simulink model "sedemo_ethernet"  (Simulink 7.5)
settings: Solver=VariableStepDiscrete  StartTime=0.0  StopTime=10.0  MaxStep=inf  RelTol=1e-3
PreLoadFcn:
  | MACInputSize = 25;
  | warning('off','MATLAB:divideByZero');
undefined symbols (not defined in the file or in its folder): des_subsystemblock, des_subsysteminport, des_subsystemoutport, des_subsystemsupportblock
libraries: simeventsrouting1 x30, simeventstranslate1 x26, simeventsattributes2 x16, simeventssink1 x13, simeventsserver1 x13, simeventsgenerators1 x11, simeventssignalmanage1 x9, simeventsgates1 x6, simeventsqueue1 x3, simeventsinfo x1
(part 1 of 5)
CloseFcn:
  | clear MACInputSize;
  | clear tout;
settings Model: Creator=The MathWorks Inc.
settings DataIOCC: SaveOutput=off  SaveTime=off
settings DebuggingCC: AlgebraicLoopMsg=error  SolverPrmCheckMsg=none  StrictBusMsg=Warning
settings SimEventsCC: propDiagAttribOutput=1  propDiagFcnCallOutput=1  propDiagStatOutput=0

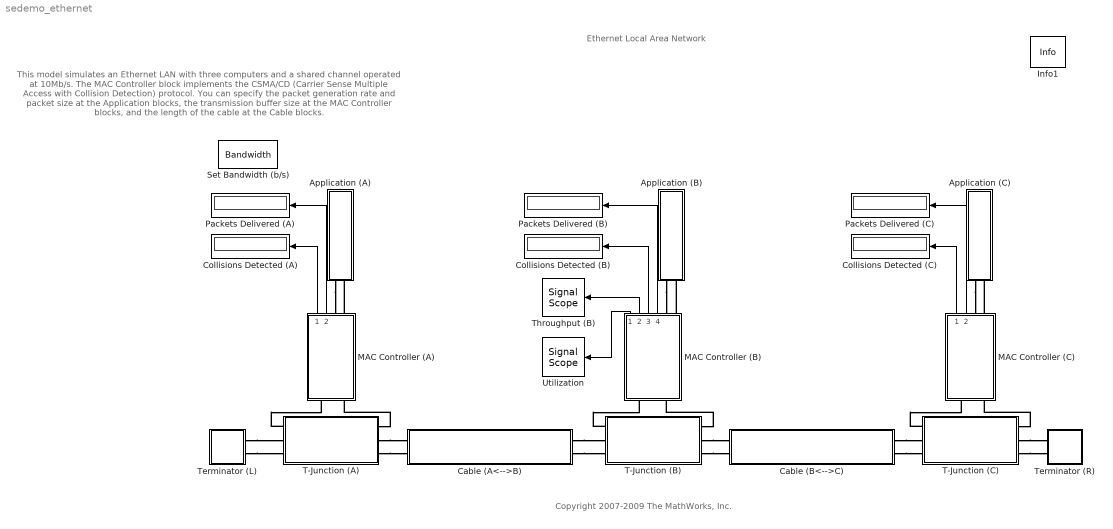
== system sedemo_ethernet ==
  note: Ethernet Local Area Network
  note: This model simulates an Ethernet LAN with three computers and a shared channel operated at 10Mb/s. The MAC Controller block implements the CSMA/CD
      | (Carrier Sense Multiple Access with Collision Detection) protocol. You can specify the packet generation rate and packet size at the Application blocks, the
      | transmission buffer size at the MAC Controller blocks, and the length of the cable at the Cable blocks.
  note: Copyright 2007-2009 The MathWorks, Inc.
  Application (A) : Subsystem  mask(Application){PacketRate=100, MinPacketSize=64, MaxPacketSize=1500, RandomSeed=678}
      mask prompts: PacketRate "Rate of packet generation (packets/s):"; MinPacketSize "Minimum packet size (bytes):"; MaxPacketSize "Maximum packet size (bytes):"; RandomSeed "Initial seed:"
      mask help: Model the generation and consumption of Ethernet data packets. Packet generation is modeled as a Poisson process. Packet size is uniformly distributed. You can specify the packet generation rate, minimum packet size and maximum packet size.
  Application (B) : Subsystem  mask(Application){PacketRate=100, MinPacketSize=64, MaxPacketSize=1500, RandomSeed=47984}
      mask prompts: PacketRate "Rate of packet generation (packets/s):"; MinPacketSize "Minimum packet size (bytes):"; MaxPacketSize "Maximum packet size (bytes):"; RandomSeed "Initial seed:"
      mask help: Model the generation and consumption of Ethernet data packets. Packet generation is modeled as a Poisson process. Packet size is uniformly distributed. You can specify the packet generation rate, minimum packet size and maximum packet size.
  Application (C) : Subsystem  mask(Application){PacketRate=100, MinPacketSize=64, MaxPacketSize=1500, RandomSeed=327278}
      mask prompts: PacketRate "Rate of packet generation (packets/s):"; MinPacketSize "Minimum packet size (bytes):"; MaxPacketSize "Maximum packet size (bytes):"; RandomSeed "Initial seed:"
      mask help: Model the generation and consumption of Ethernet data packets. Packet generation is modeled as a Poisson process. Packet size is uniformly distributed. You can specify the packet generation rate, minimum packet size and maximum packet size.
  Cable (A<-->B) : Subsystem  mask(Cable){CableLength=100}
      mask prompts: CableLength "Length (m):"
      mask help: Model the physical connection between two network terminals and the corresponding propagation delay during data transmission. You can specify the length of the cable.
  Cable (B<-->C) : Subsystem  mask(Cable){CableLength=200}
      mask prompts: CableLength "Length (m):"
      mask help: Model the physical connection between two network terminals and the corresponding propagation delay during data transmission. You can specify the length of the cable.
  "Collisions Detected (A) " : Display
  Collisions Detected (B) : Display
  Collisions Detected (C) : Display
  Info1 : simeventsinfo/Info  SystemSampleTime=-1
  MAC Controller (A) : Subsystem  mask(MAC Controller){SrcAddress=1, MACInputSize=25}
      mask prompts: SrcAddress "Source address:"; MACInputSize "Size of transmission buffer (packets):"
      mask help: Model an Ethernet controller that implements the CSMA/CD (Carrier Sense Multiple Access with Collision Detection) protocol and the binary exponential backoff algorithm. You can specify the source address of the packet and the size of the transmission buffer.
  MAC Controller (B) : Subsystem  mask(MAC Controller){SrcAddress=2, MACInputSize=25}
      mask prompts: SrcAddress "Source address:"; MACInputSize "Size of transmission buffer (packets):"
      mask help: Model an Ethernet controller that implements the CSMA/CD (Carrier Sense Multiple Access with Collision Detection) protocol and the binary exponential backoff algorithm. You can specify the source address of the packet and the size of the transmission buffer.
  MAC Controller (C) : Subsystem  mask(MAC Controller){SrcAddress=3, MACInputSize=25}
      mask prompts: SrcAddress "Source address:"; MACInputSize "Size of transmission buffer (packets):"
      mask help: Model an Ethernet controller that implements the CSMA/CD (Carrier Sense Multiple Access with Collision Detection) protocol and the binary exponential backoff algorithm. You can specify the source address of the packet and the size of the transmission buffer.
  Packets Delivered (A) : Display
  Packets Delivered (B) : Display
  Packets Delivered (C) : Display
  Set Bandwidth (b/s) : DataStoreMemory  DataStoreName=Bandwidth  InitialValue=1e7  OutDataType=sfix(16)  OutScaling=2^0
  T-Junction (A) : Subsystem
      mask Type: T-Junction
      mask Description: Connect cables from adjacent remote terminals to the local Ethernet adapter.
  T-Junction (B) : Subsystem
      mask Type: T-Junction
      mask Description: Connect cables from adjacent remote terminals to the local Ethernet adapter.
  T-Junction (C) : Subsystem
      mask Type: T-Junction
      mask Description: Connect cables from adjacent remote terminals to the local Ethernet adapter.
  Terminator (L) : Subsystem
      mask Type: Terminator
      mask Description: End an Ethernet connection.
  Terminator (R) : Subsystem
      mask Type: Terminator
      mask Description: End an Ethernet connection.
  Throughput (B) : simeventssink1/Signal Scope  Priority=1  SystemSampleTime=-1  PlotType=Stair  InputType=Signal  NumInputs=1  AttributeNameY=Count  XInputOptionSignal=Event time  XInputOptionEntity=Event time  AttributeNameX=Count  EnableEntityOutport=on  XMin=0  XMax=20  XLimitExceededOption=Stretch axis limits  YLimitExceededOption=Stretch axis limits  AxisGrid=on  AxisLegend=off  LineDisables=""  LineColors=b  LineStyles=-  LineMarkers=None  OpenScopeAtSimStart=on  Title=Throughput (kbps)  YLabel=""  XLabel=Time  FigurePosition=[635 446 386 253]  AxisZoom=off  DataStoreOption=Unlimited  DataPointsLimit=10000  StatNumberArrived=Off  ShowCountPlotted=off  ShowToolbar=on
      settings: YMin=0  YMax=1000
  Utilization : simeventssink1/Signal Scope  Priority=1  SystemSampleTime=-1  PlotType=Stair  InputType=Signal  NumInputs=1  AttributeNameY=Count  XInputOptionSignal=Event time  XInputOptionEntity=Event time  AttributeNameX=Count  EnableEntityOutport=on  XMin=0  XMax=20  XLimitExceededOption=Stretch axis limits  YLimitExceededOption=Stretch axis limits  AxisGrid=on  AxisLegend=off  LineDisables=""  LineColors=[1 0 0]  LineStyles=-  LineMarkers=None  OpenScopeAtSimStart=on  Title=Channel Utilization  YLabel=""  XLabel=Time  FigurePosition=[635 120 387 253]  AxisZoom=off  DataStoreOption=Unlimited  DataPointsLimit=10000  StatNumberArrived=Off  ShowCountPlotted=off  ShowToolbar=on
      settings: YMin=0  YMax=0.5
  wires:
  MAC Controller (A)/1(#collision) -> "Collisions Detected (A) "/1
  MAC Controller (A)/2(#success) -> Packets Delivered (A)/1
  MAC Controller (B)/3(#collision) -> Collisions Detected (B)/1
  MAC Controller (B)/4(#success) -> Packets Delivered (B)/1
  MAC Controller (B)/1(utilization) -> Utilization/1
  MAC Controller (C)/1(#collision) -> Collisions Detected (C)/1
  MAC Controller (C)/2(#success) -> Packets Delivered (C)/1
  MAC Controller (B)/2(throughput) -> Throughput (B)/1
  connections:
  Cable (B<-->C)/RConn2 -- T-Junction (C)/LConn3
  Cable (B<-->C)/RConn1 -- T-Junction (C)/LConn2
  T-Junction (B)/RConn3 -- Cable (B<-->C)/LConn2
  T-Junction (B)/RConn2 -- Cable (B<-->C)/LConn1
  T-Junction (C)/LConn1 -- MAC Controller (C)/LConn1
  T-Junction (C)/RConn1 -- MAC Controller (C)/LConn2
  T-Junction (C)/RConn2 -- Terminator (R)/LConn1
  T-Junction (C)/RConn3 -- Terminator (R)/LConn2
  MAC Controller (C)/RConn2 -- Application (C)/RConn2
  Application (C)/RConn1 -- MAC Controller (C)/RConn1
  Application (A)/RConn1 -- MAC Controller (A)/RConn1
  Cable (A<-->B)/RConn2 -- T-Junction (B)/LConn3
  Cable (A<-->B)/RConn1 -- T-Junction (B)/LConn2
  T-Junction (B)/LConn1 -- MAC Controller (B)/LConn1
  Application (B)/RConn1 -- MAC Controller (B)/RConn1
  MAC Controller (B)/RConn2 -- Application (B)/RConn2
  T-Junction (B)/RConn1 -- MAC Controller (B)/LConn2
  MAC Controller (A)/RConn2 -- Application (A)/RConn2
  Terminator (L)/LConn2 -- T-Junction (A)/LConn3
  Terminator (L)/LConn1 -- T-Junction (A)/LConn2
  T-Junction (A)/RConn3 -- Cable (A<-->B)/LConn2
  T-Junction (A)/RConn2 -- Cable (A<-->B)/LConn1
  T-Junction (A)/RConn1 -- MAC Controller (A)/LConn2
  T-Junction (A)/LConn1 -- MAC Controller (A)/LConn1

== system sedemo_ethernet/Application (A) ==
  note: Network Application
  Compute comm delay : Subsystem  LoadFcn=des_subsystemblock(gcb, 'load');  InitFcn=des_subsystemblock(gcb, 'init');  StartFcn=des_subsystemblock(gcb, 'start');  StopFcn=des_subsystemblock(gcb, 'stop');
      settings: CopyFcn=des_subsystemblock(gcb, 'copy');  DeleteFcn=des_subsystemblock(gcb, 'delete');  UndoDeleteFcn=des_subsystemblock(gcb, 'undodelete');  ModelCloseFcn=des_subsystemblock(gcb, 'modelclose');  PreSaveFcn=des_subsystemblock(gcb, 'presave');  NameChangeFcn=des_subsystemblock(gcb, 'namechange');  ParentCloseFcn=des_subsystemblock(gcb, 'parentclose');  ErrorFcn=des_error_redirect
  Data User : simeventssink1/Entity Sink  Priority=1  SystemSampleTime=-1  AvailableForArrivals=on  StatNumberArrived=Off
  Event-Based Random Number1 : simeventsgenerators1/Signal Generators/Event-Based Random Number  SystemSampleTime=-1  distribution=Uniform  meanExp=1/PacketRate  minUnif=MinPacketSize*8  maxUnif=MaxPacketSize*8  pOneBern=0.25  pSuccessBino=0.5  numTrialBino=1  meanNorm=0  stdNorm=1  minTri=1  maxTri=3  modeTri=2  thresholdLogn=0  scaleLogn=1  shapeLogn=1  pSuccessGeo=0.5  meanPoiss=1  thresholdLogl=0  scaleLogl=1  thresholdGam=0  scaleGam=1  shapeGam=1  minBeta=0  maxBeta=1  shape1Beta=1  shape2Beta=1  minUnid=0  maxUnid=1  numValueUnid=2  thresholdWbl=0  scaleWbl=1  shapeWbl=1  valueVecCont=[0 1]  cdfVecCont=[0 1]  valueVecDisc=[0 1]  probVecDisc=[0.5 0.5]  seed=RandomSeed+12345  IsProcessed=on  isConnected=1
  Event-Based Random Number2 : simeventsgenerators1/Signal Generators/Event-Based Random Number  SystemSampleTime=-1  distribution=Exponential  meanExp=1/PacketRate  minUnif=MinPacketSize  maxUnif=MaxPacketSize  pOneBern=0.25  pSuccessBino=0.5  numTrialBino=1  meanNorm=0  stdNorm=1  minTri=1  maxTri=3  modeTri=2  thresholdLogn=0  scaleLogn=1  shapeLogn=1  pSuccessGeo=0.5  meanPoiss=1  thresholdLogl=0  scaleLogl=1  thresholdGam=0  scaleGam=1  shapeGam=1  minBeta=0  maxBeta=1  shape1Beta=1  shape2Beta=1  minUnid=0  maxUnid=1  numValueUnid=2  thresholdWbl=0  scaleWbl=1  shapeWbl=1  valueVecCont=[0 1]  cdfVecCont=[0 1]  valueVecDisc=[0 1]  probVecDisc=[0.5 0.5]  seed=RandomSeed  IsProcessed=on  isConnected=1
  Set Attribute (Set packet size and comm delay) : simeventsattributes2/Set Attribute  Priority=1  DialogController=des_ddg_create  DialogControllerArgs=DataTag9  SystemSampleTime=-1  AttributeFrom=Signal port|Signal port  AttributeName=PacketSize|ServiceTime  AttributeTreatAsVector=1|1  AttributeValue=0.1|0  AttributeCreate=on  StatNumberDeparted=On  EvaluatedAttributeValue={[];[]}
  Signal Latch : simeventssignalmanage1/Signal Latch  Priority=1  SystemSampleTime=-1  InitialMemoryValue=512  WriteMemoryUpon=Change in signal from port wvc  MemoryWriteEdgeOption=Rising  SpecifyWriteEventPriority=off  PriorityMemoryWrite=7100  ReadMemoryUpon=Write to memory event  MemoryReadEdgeOption=Falling  SpecifyReadEventPriority=on  PriorityMemoryRead=7000  ReportMemoryState=off  ReportMemoryUponWrite=off  ReportMemoryUponRead=on
  Time-Based Entity Generator : simeventsgenerators1/Entity Generators/Time-Based Entity Generator  Priority=1  DialogController=des_ddg_create  DialogControllerArgs=DataTag12  SystemSampleTime=-1  GenerateEntitiesUpon=Intergeneration time from port t  Distribution=Constant  Minimum=0  Maximum=1  Mean=1/PacketRate  InitialSeed=2  Period=0.01  PriorityEntityGeneration=300  GenerateEntityAtSimulationStart=off  ResponseWhenBlocked=Pause generation  ResponseWhenUnblocked=Immediate restart  EntityType=Standard  StatNumberDeparted=Off  StatPendingEntity=Off  StatAverageIntergenerationTime=Off
  OUT : PMIOPort  Port=1  Side=Right
  IN : PMIOPort  Port=2  Side=Right
  wires:
  Compute comm delay/1(delay) -> Set Attribute (Set packet size and comm delay)/2
  Signal Latch/1 -> Compute comm delay/1(size), Set Attribute (Set packet size and comm delay)/1
  Event-Based Random Number1/1 -> Signal Latch/2
  Set Attribute (Set packet size and comm delay)/1 -> Signal Latch/1
  Event-Based Random Number2/1 -> Time-Based Entity Generator/1
  connections:
  IN/RConn1 -- Data User/LConn1
  OUT/RConn1 -- Set Attribute (Set packet size and comm delay)/RConn1
  Time-Based Entity Generator/RConn1 -- Set Attribute (Set packet size and comm delay)/LConn1

== system sedemo_ethernet/Application (B) ==
  note: Network Application
  Compute comm delay : Subsystem  LoadFcn=des_subsystemblock(gcb, 'load');  InitFcn=des_subsystemblock(gcb, 'init');  StartFcn=des_subsystemblock(gcb, 'start');  StopFcn=des_subsystemblock(gcb, 'stop');
      settings: CopyFcn=des_subsystemblock(gcb, 'copy');  DeleteFcn=des_subsystemblock(gcb, 'delete');  UndoDeleteFcn=des_subsystemblock(gcb, 'undodelete');  ModelCloseFcn=des_subsystemblock(gcb, 'modelclose');  PreSaveFcn=des_subsystemblock(gcb, 'presave');  NameChangeFcn=des_subsystemblock(gcb, 'namechange');  ParentCloseFcn=des_subsystemblock(gcb, 'parentclose');  ErrorFcn=des_error_redirect
  Data User : simeventssink1/Entity Sink  Priority=1  SystemSampleTime=-1  AvailableForArrivals=on  StatNumberArrived=Off
  Event-Based Random Number1 : simeventsgenerators1/Signal Generators/Event-Based Random Number  SystemSampleTime=-1  distribution=Uniform  meanExp=1/PacketRate  minUnif=MinPacketSize*8  maxUnif=MaxPacketSize*8  pOneBern=0.25  pSuccessBino=0.5  numTrialBino=1  meanNorm=0  stdNorm=1  minTri=1  maxTri=3  modeTri=2  thresholdLogn=0  scaleLogn=1  shapeLogn=1  pSuccessGeo=0.5  meanPoiss=1  thresholdLogl=0  scaleLogl=1  thresholdGam=0  scaleGam=1  shapeGam=1  minBeta=0  maxBeta=1  shape1Beta=1  shape2Beta=1  minUnid=0  maxUnid=1  numValueUnid=2  thresholdWbl=0  scaleWbl=1  shapeWbl=1  valueVecCont=[0 1]  cdfVecCont=[0 1]  valueVecDisc=[0 1]  probVecDisc=[0.5 0.5]  seed=RandomSeed+12345  IsProcessed=on  isConnected=1
  Event-Based Random Number2 : simeventsgenerators1/Signal Generators/Event-Based Random Number  SystemSampleTime=-1  distribution=Exponential  meanExp=1/PacketRate  minUnif=MinPacketSize  maxUnif=MaxPacketSize  pOneBern=0.25  pSuccessBino=0.5  numTrialBino=1  meanNorm=0  stdNorm=1  minTri=1  maxTri=3  modeTri=2  thresholdLogn=0  scaleLogn=1  shapeLogn=1  pSuccessGeo=0.5  meanPoiss=1  thresholdLogl=0  scaleLogl=1  thresholdGam=0  scaleGam=1  shapeGam=1  minBeta=0  maxBeta=1  shape1Beta=1  shape2Beta=1  minUnid=0  maxUnid=1  numValueUnid=2  thresholdWbl=0  scaleWbl=1  shapeWbl=1  valueVecCont=[0 1]  cdfVecCont=[0 1]  valueVecDisc=[0 1]  probVecDisc=[0.5 0.5]  seed=RandomSeed  IsProcessed=on  isConnected=1
  Set Attribute (Set packet size and comm delay) : simeventsattributes2/Set Attribute  Priority=1  DialogController=des_ddg_create  DialogControllerArgs=DataTag22  SystemSampleTime=-1  AttributeFrom=Signal port|Signal port  AttributeName=PacketSize|ServiceTime  AttributeTreatAsVector=1|1  AttributeValue=0.1|0  AttributeCreate=on  StatNumberDeparted=On  EvaluatedAttributeValue={[];[]}
  Signal Latch : simeventssignalmanage1/Signal Latch  Priority=1  SystemSampleTime=-1  InitialMemoryValue=512  WriteMemoryUpon=Change in signal from port wvc  MemoryWriteEdgeOption=Rising  SpecifyWriteEventPriority=off  PriorityMemoryWrite=7100  ReadMemoryUpon=Write to memory event  MemoryReadEdgeOption=Falling  SpecifyReadEventPriority=on  PriorityMemoryRead=7000  ReportMemoryState=off  ReportMemoryUponWrite=off  ReportMemoryUponRead=on
  Time-Based Entity Generator : simeventsgenerators1/Entity Generators/Time-Based Entity Generator  Priority=1  DialogController=des_ddg_create  DialogControllerArgs=DataTag25  SystemSampleTime=-1  GenerateEntitiesUpon=Intergeneration time from port t  Distribution=Constant  Minimum=0  Maximum=1  Mean=1/PacketRate  InitialSeed=2  Period=0.01  PriorityEntityGeneration=300  GenerateEntityAtSimulationStart=off  ResponseWhenBlocked=Pause generation  ResponseWhenUnblocked=Immediate restart  EntityType=Standard  StatNumberDeparted=Off  StatPendingEntity=Off  StatAverageIntergenerationTime=Off
  OUT : PMIOPort  Port=1  Side=Right
  IN : PMIOPort  Port=2  Side=Right
  wires:
  Event-Based Random Number2/1 -> Time-Based Entity Generator/1
  Set Attribute (Set packet size and comm delay)/1 -> Signal Latch/1
  Event-Based Random Number1/1 -> Signal Latch/2
  Signal Latch/1 -> Compute comm delay/1(size), Set Attribute (Set packet size and comm delay)/1
  Compute comm delay/1(delay) -> Set Attribute (Set packet size and comm delay)/2
  connections:
  Time-Based Entity Generator/RConn1 -- Set Attribute (Set packet size and comm delay)/LConn1
  OUT/RConn1 -- Set Attribute (Set packet size and comm delay)/RConn1
  IN/RConn1 -- Data User/LConn1

== system sedemo_ethernet/Application (C) ==
  note: Network Application
  Compute comm delay : Subsystem  LoadFcn=des_subsystemblock(gcb, 'load');  InitFcn=des_subsystemblock(gcb, 'init');  StartFcn=des_subsystemblock(gcb, 'start');  StopFcn=des_subsystemblock(gcb, 'stop');
      settings: CopyFcn=des_subsystemblock(gcb, 'copy');  DeleteFcn=des_subsystemblock(gcb, 'delete');  UndoDeleteFcn=des_subsystemblock(gcb, 'undodelete');  ModelCloseFcn=des_subsystemblock(gcb, 'modelclose');  PreSaveFcn=des_subsystemblock(gcb, 'presave');  NameChangeFcn=des_subsystemblock(gcb, 'namechange');  ParentCloseFcn=des_subsystemblock(gcb, 'parentclose');  ErrorFcn=des_error_redirect
  Data User : simeventssink1/Entity Sink  Priority=1  SystemSampleTime=-1  AvailableForArrivals=on  StatNumberArrived=Off
  Event-Based Random Number1 : simeventsgenerators1/Signal Generators/Event-Based Random Number  SystemSampleTime=-1  distribution=Uniform  meanExp=1/PacketRate  minUnif=MinPacketSize*8  maxUnif=MaxPacketSize*8  pOneBern=0.25  pSuccessBino=0.5  numTrialBino=1  meanNorm=0  stdNorm=1  minTri=1  maxTri=3  modeTri=2  thresholdLogn=0  scaleLogn=1  shapeLogn=1  pSuccessGeo=0.5  meanPoiss=1  thresholdLogl=0  scaleLogl=1  thresholdGam=0  scaleGam=1  shapeGam=1  minBeta=0  maxBeta=1  shape1Beta=1  shape2Beta=1  minUnid=0  maxUnid=1  numValueUnid=2  thresholdWbl=0  scaleWbl=1  shapeWbl=1  valueVecCont=[0 1]  cdfVecCont=[0 1]  valueVecDisc=[0 1]  probVecDisc=[0.5 0.5]  seed=RandomSeed+12345  IsProcessed=on  isConnected=1
  Event-Based Random Number2 : simeventsgenerators1/Signal Generators/Event-Based Random Number  SystemSampleTime=-1  distribution=Exponential  meanExp=1/PacketRate  minUnif=MinPacketSize  maxUnif=MaxPacketSize  pOneBern=0.25  pSuccessBino=0.5  numTrialBino=1  meanNorm=0  stdNorm=1  minTri=1  maxTri=3  modeTri=2  thresholdLogn=0  scaleLogn=1  shapeLogn=1  pSuccessGeo=0.5  meanPoiss=1  thresholdLogl=0  scaleLogl=1  thresholdGam=0  scaleGam=1  shapeGam=1  minBeta=0  maxBeta=1  shape1Beta=1  shape2Beta=1  minUnid=0  maxUnid=1  numValueUnid=2  thresholdWbl=0  scaleWbl=1  shapeWbl=1  valueVecCont=[0 1]  cdfVecCont=[0 1]  valueVecDisc=[0 1]  probVecDisc=[0.5 0.5]  seed=RandomSeed  IsProcessed=on  isConnected=1
  Set Attribute (Set packet size and comm delay) : simeventsattributes2/Set Attribute  Priority=1  DialogController=des_ddg_create  DialogControllerArgs=DataTag35  SystemSampleTime=-1  AttributeFrom=Signal port|Signal port  AttributeName=PacketSize|ServiceTime  AttributeTreatAsVector=1|1  AttributeValue=0.1|0  AttributeCreate=on  StatNumberDeparted=On  EvaluatedAttributeValue={[];[]}
  Signal Latch : simeventssignalmanage1/Signal Latch  Priority=1  SystemSampleTime=-1  InitialMemoryValue=512  WriteMemoryUpon=Change in signal from port wvc  MemoryWriteEdgeOption=Rising  SpecifyWriteEventPriority=off  PriorityMemoryWrite=7100  ReadMemoryUpon=Write to memory event  MemoryReadEdgeOption=Falling  SpecifyReadEventPriority=on  PriorityMemoryRead=7000  ReportMemoryState=off  ReportMemoryUponWrite=off  ReportMemoryUponRead=on
  Time-Based Entity Generator : simeventsgenerators1/Entity Generators/Time-Based Entity Generator  Priority=1  DialogController=des_ddg_create  DialogControllerArgs=DataTag38  SystemSampleTime=-1  GenerateEntitiesUpon=Intergeneration time from port t  Distribution=Constant  Minimum=0  Maximum=1  Mean=1/PacketRate  InitialSeed=2  Period=0.01  PriorityEntityGeneration=300  GenerateEntityAtSimulationStart=off  ResponseWhenBlocked=Pause generation  ResponseWhenUnblocked=Immediate restart  EntityType=Standard  StatNumberDeparted=Off  StatPendingEntity=Off  StatAverageIntergenerationTime=Off
  OUT : PMIOPort  Port=1  Side=Right
  IN : PMIOPort  Port=2  Side=Right
  wires:
  Compute comm delay/1(delay) -> Set Attribute (Set packet size and comm delay)/2
  Signal Latch/1 -> Compute comm delay/1(size), Set Attribute (Set packet size and comm delay)/1
  Event-Based Random Number1/1 -> Signal Latch/2
  Set Attribute (Set packet size and comm delay)/1 -> Signal Latch/1
  Event-Based Random Number2/1 -> Time-Based Entity Generator/1
  connections:
  IN/RConn1 -- Data User/LConn1
  OUT/RConn1 -- Set Attribute (Set packet size and comm delay)/RConn1
  Time-Based Entity Generator/RConn1 -- Set Attribute (Set packet size and comm delay)/LConn1

== system sedemo_ethernet/Cable (A<-->B) ==
  note: Network Cable
  Infinite Server 1 : simeventsserver1/Infinite Server  Priority=1  SystemSampleTime=-1  ServiceTimeFrom=Dialog  ServiceTime=CableLength/3e8  AttributeName=ServiceTime  PriorityServiceCompletion=500  EnableTOPort=off  StatNumberDeparted=Off  StatNumberInBlock=Off  StatPendingEntity=Off  StatNumberPending=Off  StatAverageWait=Off  StatNumberTimedout=Off
  Infinite Server 2 : simeventsserver1/Infinite Server  Priority=1  SystemSampleTime=-1  ServiceTimeFrom=Dialog  ServiceTime=CableLength/3e8  AttributeName=ServiceTime  PriorityServiceCompletion=500  EnableTOPort=off  StatNumberDeparted=Off  StatNumberInBlock=Off  StatPendingEntity=Off  StatNumberPending=Off  StatAverageWait=Off  StatNumberTimedout=Off
  IN_L : PMIOPort  Port=1  Side=Left
  OUT_R : PMIOPort  Port=2  Side=Right
  IN_R : PMIOPort  Port=3  Side=Right
  OUT_L : PMIOPort  Port=4  Side=Left
  connections:
  IN_L/RConn1 -- Infinite Server 1/LConn1
  OUT_R/RConn1 -- Infinite Server 1/RConn1
  IN_R/RConn1 -- Infinite Server 2/LConn1
  OUT_L/RConn1 -- Infinite Server 2/RConn1

== system sedemo_ethernet/Cable (B<-->C) ==
  note: Network Cable
  Infinite Server 1 : simeventsserver1/Infinite Server  Priority=1  SystemSampleTime=-1  ServiceTimeFrom=Dialog  ServiceTime=CableLength/3e8  AttributeName=ServiceTime  PriorityServiceCompletion=500  EnableTOPort=off  StatNumberDeparted=Off  StatNumberInBlock=Off  StatPendingEntity=Off  StatNumberPending=Off  StatAverageWait=Off  StatNumberTimedout=Off
  Infinite Server 2 : simeventsserver1/Infinite Server  Priority=1  SystemSampleTime=-1  ServiceTimeFrom=Dialog  ServiceTime=CableLength/3e8  AttributeName=ServiceTime  PriorityServiceCompletion=500  EnableTOPort=off  StatNumberDeparted=Off  StatNumberInBlock=Off  StatPendingEntity=Off  StatNumberPending=Off  StatAverageWait=Off  StatNumberTimedout=Off
  IN_L : PMIOPort  Port=1  Side=Left
  OUT_R : PMIOPort  Port=2  Side=Right
  IN_R : PMIOPort  Port=3  Side=Right
  OUT_L : PMIOPort  Port=4  Side=Left
  connections:
  OUT_L/RConn1 -- Infinite Server 2/RConn1
  IN_R/RConn1 -- Infinite Server 2/LConn1
  OUT_R/RConn1 -- Infinite Server 1/RConn1
  IN_L/RConn1 -- Infinite Server 1/LConn1

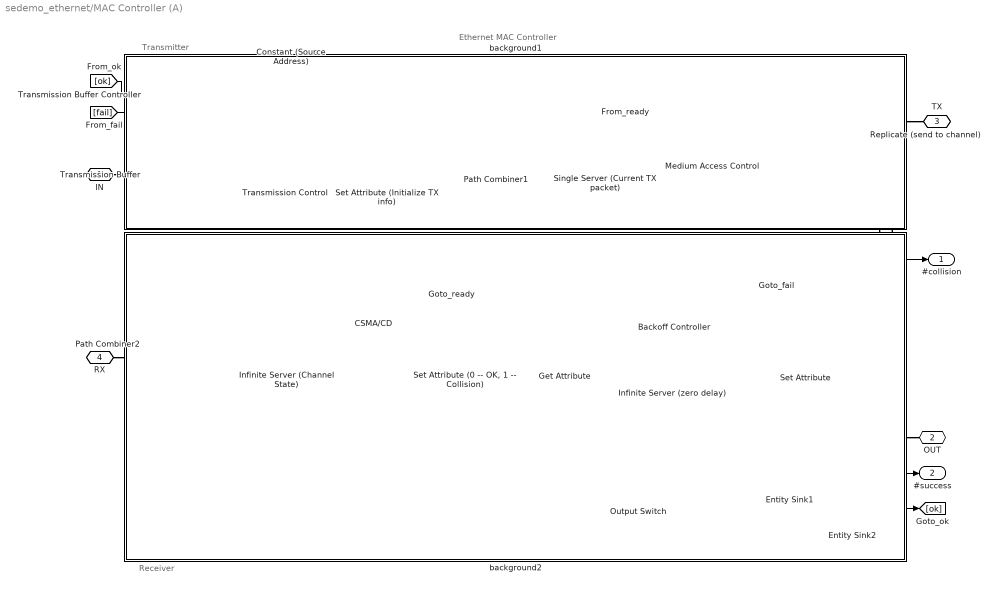
== system sedemo_ethernet/MAC Controller (A) ==
  note: Receiver
  note: Transmitter
  note: Ethernet MAC Controller
  Backoff Controller : Subsystem  LoadFcn=des_subsystemblock(gcb, 'load');  InitFcn=des_subsystemblock(gcb, 'init');  StartFcn=des_subsystemblock(gcb, 'start');  StopFcn=des_subsystemblock(gcb, 'stop');
      settings: CopyFcn=des_subsystemblock(gcb, 'copy');  DeleteFcn=des_subsystemblock(gcb, 'delete');  UndoDeleteFcn=des_subsystemblock(gcb, 'undodelete');  ModelCloseFcn=des_subsystemblock(gcb, 'modelclose');  PreSaveFcn=des_subsystemblock(gcb, 'presave');  NameChangeFcn=des_subsystemblock(gcb, 'namechange');  ParentCloseFcn=des_subsystemblock(gcb, 'parentclose');  ErrorFcn=des_error_redirect
  CSMA/CD : Subsystem
  Constant (Source Address) : Constant  Value=SrcAddress  OutDataType=sfix(16)  OutScaling=2^0
  Entity Sink1 : simeventssink1/Entity Sink  Priority=1  SystemSampleTime=-1  AvailableForArrivals=on  StatNumberArrived=On
  Entity Sink2 : simeventssink1/Entity Sink  Priority=1  SystemSampleTime=-1  AvailableForArrivals=on  StatNumberArrived=Off
  Get Attribute : simeventsattributes2/Get Attribute  Priority=1  DialogController=des_ddg_create  DialogControllerArgs=DataTag70  SystemSampleTime=-1  AttributeName=SrcAddress|NumCollision|Collision  AttributeMissing=Error|Error|Error  AttributeDefaultValue=0|0|0  AttributeSendTiming=After entity departure|After entity departure|After entity departure  AttributeTreatAsVector=1|1|1  StatNumberDeparted=Off  EvaluatedDefaultAttributeValue={[];[];[]}
  Infinite Server (Channel State) : simeventsserver1/Infinite Server  Priority=1  SystemSampleTime=-1  ServiceTimeFrom=Attribute  ServiceTime=1  AttributeName=ServiceTime  PriorityServiceCompletion=500  EnableTOPort=off  StatNumberDeparted=Off  StatNumberInBlock=On  StatPendingEntity=Off  StatNumberPending=Off  StatAverageWait=Off  StatNumberTimedout=Off
  Infinite Server (zero delay) : simeventsserver1/Infinite Server  Priority=1  SystemSampleTime=-1  ServiceTimeFrom=Dialog  ServiceTime=0  AttributeName=ServiceTime  PriorityServiceCompletion=200  EnableTOPort=off  StatNumberDeparted=Off  StatNumberInBlock=Off  StatPendingEntity=Off  StatNumberPending=Off  StatAverageWait=Off  StatNumberTimedout=Off
  Medium Access Control : simeventsgates1/Enabled Gate  Priority=1  SystemSampleTime=-1  SpecifyEventPriority=off  PriorityGateEnableOpenClose=200  StatNumberDeparted=Off
  Output Switch : simeventsrouting1/Output Switch  Priority=1  SystemSampleTime=-1  NumberOutputPorts=4  SwitchingCriterion=From attribute  InitialSeed=34567  AttributeName=Route  InitialConditionsOpt=off  InitialConditions=1  EntityBufferOpt=off  SpecifyEventPriority=off  PriorityOutputSwitchSelectPort=4100  TimeoutPortOpt=off  StatNumberDeparted=Off  StatNumberTimedOut=Off  StatPendingEntity=Off  StatLastDeparturePort=Off  EvaluatedNumPorts=4
  Path Combiner1 : simeventsrouting1/Path Combiner  Priority=1  SystemSampleTime=-1  NumberInputPorts=2  InputPortPrecedence=IN1 port  InitialSeed=45675  SpecifyEventPriority=off  PriorityPathCombinerPortPrecedenceSelection=4100  StatNumberDeparted=Off  StatLastArrivalPort=Off  EvaluatedNumPorts=2
  Path Combiner2 : simeventsrouting1/Path Combiner  Priority=1  SystemSampleTime=-1  NumberInputPorts=2  InputPortPrecedence=IN1 port  InitialSeed=45675  SpecifyEventPriority=off  PriorityPathCombinerPortPrecedenceSelection=4100  StatNumberDeparted=Off  StatLastArrivalPort=Off  EvaluatedNumPorts=2
  Replicate (send to channel) : simeventsrouting1/Replicate  Priority=1  SystemSampleTime=-1  NumberOutputPorts=2  ReplicateEntityWhen=All entity output ports are not blocked  OutputPortPrecedence=OUT1 port  InitialSeed=56789  ActionUponBlocking=Discard entity  StatNumberArrived=Off  StatNumberDeparted=Off  EvaluatedNumPorts=2
  Set Attribute : simeventsattributes2/Set Attribute  Priority=1  DialogController=des_ddg_create  DialogControllerArgs=DataTag79  SystemSampleTime=-1  AttributeFrom=Signal port|Signal port|Signal port  AttributeName=Route|NumCollision|BckoffTime  AttributeTreatAsVector=1|1|1  AttributeValue=0|0|0  AttributeCreate=on  StatNumberDeparted=Off  EvaluatedAttributeValue={[];[];[]}
  "Set Attribute (0 -- OK, 1 -- Collision)" : simeventsattributes2/Set Attribute  Priority=1  DialogController=des_ddg_create  DialogControllerArgs=DataTag81  SystemSampleTime=-1  AttributeFrom=Signal port  AttributeName=Collision  AttributeTreatAsVector=1  AttributeValue=0  AttributeCreate=on  StatNumberDeparted=Off  EvaluatedAttributeValue={[]}
  Set Attribute (Initialize TX info) : simeventsattributes2/Set Attribute  Priority=1  DialogController=des_ddg_create  DialogControllerArgs=DataTag83  SystemSampleTime=-1  AttributeFrom=Signal port|Dialog|Dialog  AttributeName=SrcAddress|BckoffTime|NumCollision  AttributeTreatAsVector=1|1|1  AttributeValue=0|0|0  AttributeCreate=on  StatNumberDeparted=Off  EvaluatedAttributeValue={[];0;0}
  Single Server (Current TX packet) : simeventsserver1/Single Server  Priority=1  SystemSampleTime=-1  ServiceTimeFrom=Attribute  ServiceTime=0  AttributeName=BckoffTime  PriorityServiceCompletion=500  PermitPreemption=off  SortingAttributeName=PriorityAttributeName  SortingDirection=Ascending  WriteToAttribute=off  ResidualAttributeName=ResidualServiceTime  CreateAttribute=on  EnableTOPort=off  StatNumberDeparted=Off  StatNumberInBlock=Off  StatNumberPreempted=Off  StatPendingEntity=Off  StatAverageWait=Off  StatUtilization=Off  StatNumberTimedout=Off
  Transmission Buffer : simeventsqueue1/FIFO Queue  Priority=1  SystemSampleTime=-1  Capacity=MACInputSize  EnableTOPort=off  StatNumberDeparted=Off  StatNumberInBlock=Off  StatPendingEntity=Off  StatAverageWait=Off  StatAverageQueueLength=Off  StatNumberTimedout=Off
  Transmission Buffer Controller : Subsystem
  Transmission Control : simeventsgates1/Enabled Gate  Priority=1  SystemSampleTime=-1  SpecifyEventPriority=off  PriorityGateEnableOpenClose=200  StatNumberDeparted=On
  background1 : Subsystem
      mask Display: disp('')
  background2 : Subsystem
      mask Display: disp('')
  IN : PMIOPort  Port=1  Side=Right
  OUT : PMIOPort  Port=2  Side=Right
  TX : PMIOPort  Port=3  Side=Left
  RX : PMIOPort  Port=4  Side=Left
  #collision : Outport  OutDataType=sfix(16)  OutScaling=2^0
  #success : Outport  Port=2  OutDataType=sfix(16)  OutScaling=2^0
  wires:
  [ok] -> Transmission Buffer Controller/2(#success)
  [fail] -> Transmission Buffer Controller/3(#failure)
  Backoff Controller/2(#failure) -> [fail]
  [rdy] -> Medium Access Control/1
  CSMA/CD/1(l_ready) -> [rdy]
  Transmission Control/1 -> Transmission Buffer Controller/1(#tx)
  Infinite Server (Channel State)/1 -> CSMA/CD/1(l_status)
  Entity Sink1/1 -> [ok], #success/1
  CSMA/CD/2(pck_ok) -> "Set Attribute (0 -- OK, 1 -- Collision)"/1
  Transmission Buffer Controller/1(state) -> Transmission Control/1
  Constant (Source Address)/1 -> Set Attribute (Initialize TX info)/1
  Get Attribute/1 -> Backoff Controller/1(SrcAddr)
  Get Attribute/3 -> Backoff Controller/3(collision)
  Get Attribute/2 -> Backoff Controller/2(#collision)
  Backoff Controller/1(#sum) -> #collision/1
  Backoff Controller/5(bckoffTime) -> Set Attribute/3
  Backoff Controller/4(#collision1) -> Set Attribute/2
  Backoff Controller/3(route) -> Set Attribute/1
  connections:
  Output Switch/RConn1 -- OUT/RConn1
  Single Server (Current TX packet)/RConn1 -- Medium Access Control/LConn1
  Path Combiner2/RConn1 -- Infinite Server (Channel State)/LConn1
  Infinite Server (Channel State)/RConn1 -- "Set Attribute (0 -- OK, 1 -- Collision)"/LConn1
  IN/RConn1 -- Transmission Buffer/LConn1
  Medium Access Control/RConn1 -- Replicate (send to channel)/LConn1
  RX/RConn1 -- Path Combiner2/LConn2
  Path Combiner1/RConn1 -- Single Server (Current TX packet)/LConn1
  Replicate (send to channel)/RConn2 -- Path Combiner2/LConn1
  Transmission Buffer/RConn1 -- Transmission Control/LConn1
  Replicate (send to channel)/RConn1 -- TX/RConn1
  Set Attribute (Initialize TX info)/RConn1 -- Path Combiner1/LConn2
  Transmission Control/RConn1 -- Set Attribute (Initialize TX info)/LConn1
  Output Switch/RConn3 -- Entity Sink2/LConn1
  Output Switch/RConn2 -- Entity Sink1/LConn1
  Get Attribute/RConn1 -- Infinite Server (zero delay)/LConn1
  Infinite Server (zero delay)/RConn1 -- Set Attribute/LConn1
  "Set Attribute (0 -- OK, 1 -- Collision)"/RConn1 -- Get Attribute/LConn1
  Set Attribute/RConn1 -- Output Switch/LConn1
  Output Switch/RConn4 -- Path Combiner1/LConn1

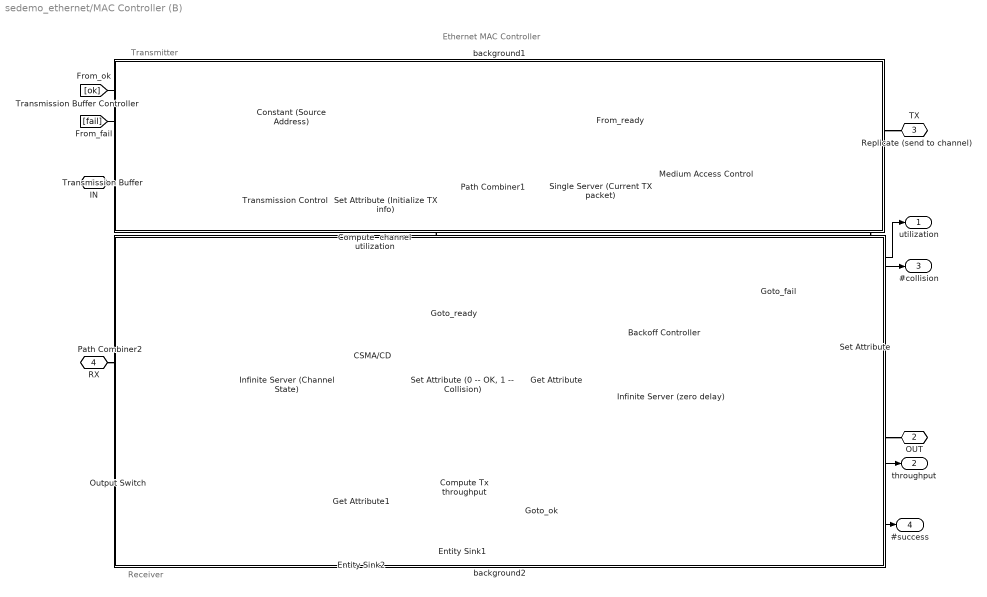
== system sedemo_ethernet/MAC Controller (B) ==
  note: Receiver
  note: Transmitter
  note: Ethernet MAC Controller
  Backoff Controller : Subsystem  LoadFcn=des_subsystemblock(gcb, 'load');  InitFcn=des_subsystemblock(gcb, 'init');  StartFcn=des_subsystemblock(gcb, 'start');  StopFcn=des_subsystemblock(gcb, 'stop');
      settings: CopyFcn=des_subsystemblock(gcb, 'copy');  DeleteFcn=des_subsystemblock(gcb, 'delete');  UndoDeleteFcn=des_subsystemblock(gcb, 'undodelete');  ModelCloseFcn=des_subsystemblock(gcb, 'modelclose');  PreSaveFcn=des_subsystemblock(gcb, 'presave');  NameChangeFcn=des_subsystemblock(gcb, 'namechange');  ParentCloseFcn=des_subsystemblock(gcb, 'parentclose');  ErrorFcn=des_error_redirect
  CSMA/CD : Subsystem
  Compute  channel utilization : Subsystem  LoadFcn=des_subsystemblock(gcb, 'load');  InitFcn=des_subsystemblock(gcb, 'init');  StartFcn=des_subsystemblock(gcb, 'start');  StopFcn=des_subsystemblock(gcb, 'stop');
      settings: CopyFcn=des_subsystemblock(gcb, 'copy');  DeleteFcn=des_subsystemblock(gcb, 'delete');  UndoDeleteFcn=des_subsystemblock(gcb, 'undodelete');  ModelCloseFcn=des_subsystemblock(gcb, 'modelclose');  PreSaveFcn=des_subsystemblock(gcb, 'presave');  NameChangeFcn=des_subsystemblock(gcb, 'namechange');  ParentCloseFcn=des_subsystemblock(gcb, 'parentclose');  ErrorFcn=des_error_redirect
  Compute Tx throughput : Subsystem  LoadFcn=des_subsystemblock(gcb, 'load');  InitFcn=des_subsystemblock(gcb, 'init');  StartFcn=des_subsystemblock(gcb, 'start');  StopFcn=des_subsystemblock(gcb, 'stop');
      settings: CopyFcn=des_subsystemblock(gcb, 'copy');  DeleteFcn=des_subsystemblock(gcb, 'delete');  UndoDeleteFcn=des_subsystemblock(gcb, 'undodelete');  ModelCloseFcn=des_subsystemblock(gcb, 'modelclose');  PreSaveFcn=des_subsystemblock(gcb, 'presave');  NameChangeFcn=des_subsystemblock(gcb, 'namechange');  ParentCloseFcn=des_subsystemblock(gcb, 'parentclose');  ErrorFcn=des_error_redirect
  Constant (Source Address) : Constant  Value=SrcAddress  OutDataType=sfix(16)  OutScaling=2^0
  Entity Sink1 : simeventssink1/Entity Sink  Priority=1  SystemSampleTime=-1  AvailableForArrivals=on  StatNumberArrived=On
  Entity Sink2 : simeventssink1/Entity Sink  Priority=1  SystemSampleTime=-1  AvailableForArrivals=on  StatNumberArrived=Off
  Get Attribute : simeventsattributes2/Get Attribute  Priority=1  DialogController=des_ddg_create  DialogControllerArgs=DataTag139  SystemSampleTime=-1  AttributeName=SrcAddress|NumCollision|Collision  AttributeMissing=Error|Error|Error  AttributeDefaultValue=0|0|0  AttributeSendTiming=After entity departure|After entity departure|After entity departure  AttributeTreatAsVector=1|1|1  StatNumberDeparted=Off  EvaluatedDefaultAttributeValue={[];[];[]}
  Get Attribute1 : simeventsattributes2/Get Attribute  Priority=1  DialogController=des_ddg_create  DialogControllerArgs=DataTag141  SystemSampleTime=-1  AttributeName=PacketSize  AttributeMissing=Error  AttributeDefaultValue=0  AttributeSendTiming=After entity departure  AttributeTreatAsVector=1  StatNumberDeparted=Off  EvaluatedDefaultAttributeValue={[]}
  Infinite Server (Channel State) : simeventsserver1/Infinite Server  Priority=1  SystemSampleTime=-1  ServiceTimeFrom=Attribute  ServiceTime=1  AttributeName=ServiceTime  PriorityServiceCompletion=500  EnableTOPort=off  StatNumberDeparted=Off  StatNumberInBlock=On  StatPendingEntity=Off  StatNumberPending=Off  StatAverageWait=Off  StatNumberTimedout=Off
  Infinite Server (zero delay) : simeventsserver1/Infinite Server  Priority=1  SystemSampleTime=-1  ServiceTimeFrom=Dialog  ServiceTime=0  AttributeName=ServiceTime  PriorityServiceCompletion=200  EnableTOPort=off  StatNumberDeparted=Off  StatNumberInBlock=Off  StatPendingEntity=Off  StatNumberPending=Off  StatAverageWait=Off  StatNumberTimedout=Off
  Medium Access Control : simeventsgates1/Enabled Gate  Priority=1  SystemSampleTime=-1  SpecifyEventPriority=off  PriorityGateEnableOpenClose=200  StatNumberDeparted=Off
  Output Switch : simeventsrouting1/Output Switch  Priority=1  SystemSampleTime=-1  NumberOutputPorts=4  SwitchingCriterion=From attribute  InitialSeed=34567  AttributeName=Route  InitialConditionsOpt=off  InitialConditions=1  EntityBufferOpt=off  SpecifyEventPriority=off  PriorityOutputSwitchSelectPort=4100  TimeoutPortOpt=off  StatNumberDeparted=Off  StatNumberTimedOut=Off  StatPendingEntity=Off  StatLastDeparturePort=Off  EvaluatedNumPorts=4
  Path Combiner1 : simeventsrouting1/Path Combiner  Priority=1  SystemSampleTime=-1  NumberInputPorts=2  InputPortPrecedence=IN1 port  InitialSeed=45675  SpecifyEventPriority=off  PriorityPathCombinerPortPrecedenceSelection=4100  StatNumberDeparted=Off  StatLastArrivalPort=Off  EvaluatedNumPorts=2
  Path Combiner2 : simeventsrouting1/Path Combiner  Priority=1  SystemSampleTime=-1  NumberInputPorts=2  InputPortPrecedence=IN1 port  InitialSeed=45675  SpecifyEventPriority=off  PriorityPathCombinerPortPrecedenceSelection=4100  StatNumberDeparted=Off  StatLastArrivalPort=Off  EvaluatedNumPorts=2
  Replicate (send to channel) : simeventsrouting1/Replicate  Priority=1  SystemSampleTime=-1  NumberOutputPorts=2  ReplicateEntityWhen=All entity output ports are not blocked  OutputPortPrecedence=OUT1 port  InitialSeed=56789  ActionUponBlocking=Discard entity  StatNumberArrived=Off  StatNumberDeparted=Off  EvaluatedNumPorts=2
  Set Attribute : simeventsattributes2/Set Attribute  Priority=1  DialogController=des_ddg_create  DialogControllerArgs=DataTag150  SystemSampleTime=-1  AttributeFrom=Signal port|Signal port|Signal port  AttributeName=Route|NumCollision|BckoffTime  AttributeTreatAsVector=1|1|1  AttributeValue=0|0|0  AttributeCreate=on  StatNumberDeparted=Off  EvaluatedAttributeValue={[];[];[]}
  "Set Attribute (0 -- OK, 1 -- Collision)" : simeventsattributes2/Set Attribute  Priority=1  DialogController=des_ddg_create  DialogControllerArgs=DataTag152  SystemSampleTime=-1  AttributeFrom=Signal port  AttributeName=Collision  AttributeTreatAsVector=1  AttributeValue=0  AttributeCreate=on  StatNumberDeparted=Off  EvaluatedAttributeValue={[]}
  Set Attribute (Initialize TX info) : simeventsattributes2/Set Attribute  Priority=1  DialogController=des_ddg_create  DialogControllerArgs=DataTag154  SystemSampleTime=-1  AttributeFrom=Signal port|Dialog|Dialog  AttributeName=SrcAddress|BckoffTime|NumCollision  AttributeTreatAsVector=1|1|1  AttributeValue=0|0|0  AttributeCreate=on  StatNumberDeparted=Off  EvaluatedAttributeValue={[];0;0}
  Single Server (Current TX packet) : simeventsserver1/Single Server  Priority=1  SystemSampleTime=-1  ServiceTimeFrom=Attribute  ServiceTime=0  AttributeName=BckoffTime  PriorityServiceCompletion=500  PermitPreemption=off  SortingAttributeName=PriorityAttributeName  SortingDirection=Ascending  WriteToAttribute=off  ResidualAttributeName=ResidualServiceTime  CreateAttribute=on  EnableTOPort=off  StatNumberDeparted=Off  StatNumberInBlock=Off  StatNumberPreempted=Off  StatPendingEntity=Off  StatAverageWait=Off  StatUtilization=Off  StatNumberTimedout=Off
  Transmission Buffer : simeventsqueue1/FIFO Queue  Priority=1  SystemSampleTime=-1  Capacity=MACInputSize  EnableTOPort=off  StatNumberDeparted=Off  StatNumberInBlock=Off  StatPendingEntity=Off  StatAverageWait=Off  StatAverageQueueLength=Off  StatNumberTimedout=Off
  Transmission Buffer Controller : Subsystem
  Transmission Control : simeventsgates1/Enabled Gate  Priority=1  SystemSampleTime=-1  SpecifyEventPriority=off  PriorityGateEnableOpenClose=200  StatNumberDeparted=On
  background1 : Subsystem
      mask Display: disp('')
  background2 : Subsystem
      mask Display: disp('')
  IN : PMIOPort  Port=1  Side=Right
  OUT : PMIOPort  Port=2  Side=Right
  TX : PMIOPort  Port=3  Side=Left
  RX : PMIOPort  Port=4  Side=Left
  utilization : Outport  OutDataType=sfix(16)  OutScaling=2^0
  throughput : Outport  Port=2  OutDataType=sfix(16)  OutScaling=2^0
  #collision : Outport  Port=3  OutDataType=sfix(16)  OutScaling=2^0
  #success : Outport  Port=4  OutDataType=sfix(16)  OutScaling=2^0
  wires:
  Get Attribute/3 -> Backoff Controller/3(collision)
  Get Attribute/2 -> Backoff Controller/2(#collision)
  Backoff Controller/3(route) -> Set Attribute/1
  Backoff Controller/4(#collision1) -> Set Attribute/2
  Entity Sink1/1 -> [ok], #success/1
  Infinite Server (Channel State)/1 -> Compute  channel utilization/1(#n), CSMA/CD/1(l_status)
  [rdy] -> Medium Access Control/1
  CSMA/CD/1(l_ready) -> [rdy]
  [fail] -> Transmission Buffer Controller/3(#failure)
  Backoff Controller/2(#failure) -> [fail]
  [ok] -> Transmission Buffer Controller/2(#success)
  Compute Tx throughput/1(rate) -> throughput/1
  Get Attribute1/1 -> Compute Tx throughput/1(PckSize)
  Backoff Controller/5(bckoffTime) -> Set Attribute/3
  Backoff Controller/1(#sum) -> #collision/1
  Get Attribute/1 -> Backoff Controller/1(SrcAddr)
  Constant (Source Address)/1 -> Set Attribute (Initialize TX info)/1
  Transmission Buffer Controller/1(state) -> Transmission Control/1
  CSMA/CD/2(pck_ok) -> "Set Attribute (0 -- OK, 1 -- Collision)"/1
  Compute  channel utilization/1(util) -> utilization/1
  Transmission Control/1 -> Transmission Buffer Controller/1(#tx)
  connections:
  Get Attribute1/RConn1 -- Entity Sink1/LConn1
  Output Switch/RConn2 -- Get Attribute1/LConn1
  Output Switch/RConn4 -- Path Combiner1/LConn1
  Output Switch/RConn1 -- OUT/RConn1
  Set Attribute/RConn1 -- Output Switch/LConn1
  "Set Attribute (0 -- OK, 1 -- Collision)"/RConn1 -- Get Attribute/LConn1
  Infinite Server (zero delay)/RConn1 -- Set Attribute/LConn1
  Get Attribute/RConn1 -- Infinite Server (zero delay)/LConn1
  Output Switch/RConn3 -- Entity Sink2/LConn1
  Transmission Control/RConn1 -- Set Attribute (Initialize TX info)/LConn1
  Set Attribute (Initialize TX info)/RConn1 -- Path Combiner1/LConn2
  Replicate (send to channel)/RConn1 -- TX/RConn1
  Transmission Buffer/RConn1 -- Transmission Control/LConn1
  Replicate (send to channel)/RConn2 -- Path Combiner2/LConn1
  Path Combiner1/RConn1 -- Single Server (Current TX packet)/LConn1
  RX/RConn1 -- Path Combiner2/LConn2
  Medium Access Control/RConn1 -- Replicate (send to channel)/LConn1
  IN/RConn1 -- Transmission Buffer/LConn1
  Infinite Server (Channel State)/RConn1 -- "Set Attribute (0 -- OK, 1 -- Collision)"/LConn1
  Path Combiner2/RConn1 -- Infinite Server (Channel State)/LConn1
  Single Server (Current TX packet)/RConn1 -- Medium Access Control/LConn1
